simulink model "EstimateLaneCenter"  (R2024a)
settings: configuration reference "csMultiInstance" (kept outside this file)
undefined symbols (not defined in the file or in its folder): HalfLaneWidth, Ts
Description:
  | Model to esitmate centerline of the lane from information about the lane boundaries.
settings Model: DataDictionary=DD_EstimateLaneCenter.sldd  EnableAccessToBaseWorkspace=off  Creator=The MathWorks, Inc.  LastModifiedBy=The MathWorks, Inc.
settings ConfigSetRef: SourceName=csMultiInstance

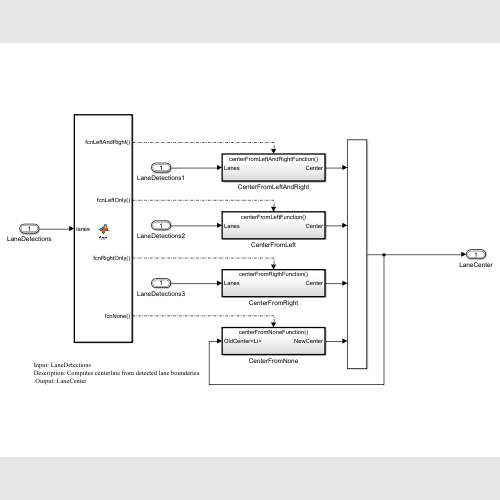
[thumbnail: Simulink's stored preview of the top-level diagram]
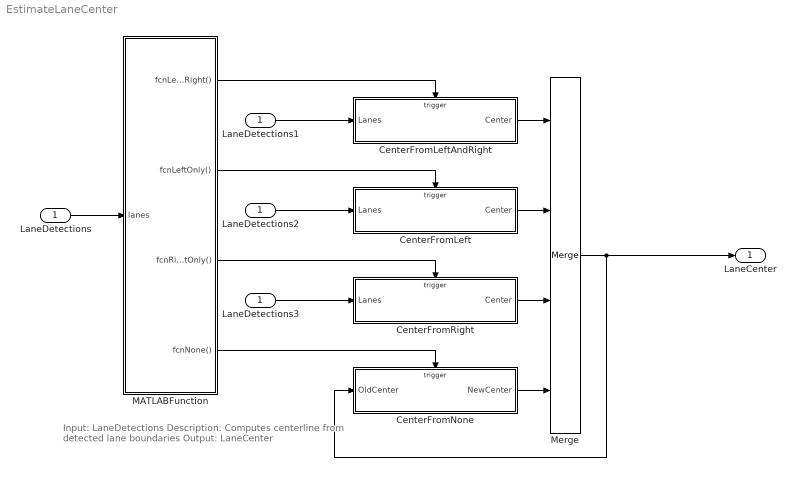
== system EstimateLaneCenter ==
  note: Input: LaneDetections
      | Description: Computes centerline from detected lane boundaries
      | Output: LaneCenter
  LaneDetections : Inport  OutDataTypeStr=Bus: LaneSensor  PortDimensions=1  SampleTime=Ts
  CenterFromLeft : Subsystem  TreatAsAtomicUnit=on
  CenterFromLeftAndRight : Subsystem  TreatAsAtomicUnit=on
  CenterFromNone : Subsystem  TreatAsAtomicUnit=on
  CenterFromRight : Subsystem  TreatAsAtomicUnit=on
  LaneDetections1 : InportShadow  OutDataTypeStr=Bus: LaneSensor  PortDimensions=1  SampleTime=Ts
  LaneDetections2 : InportShadow  OutDataTypeStr=Bus: LaneSensor  PortDimensions=1  SampleTime=Ts
  LaneDetections3 : InportShadow  OutDataTypeStr=Bus: LaneSensor  PortDimensions=1  SampleTime=Ts
  MATLABFunction : MATLAB Function  TreatAsAtomicUnit=on
  Merge : Merge  Inputs=4
  LaneCenter : Outport  OutDataTypeStr=Bus: BusLaneCenter  PortDimensions=1  SampleTime=Ts
  wires:
  MATLABFunction/1(fcnLeftAndRight()) -> CenterFromLeftAndRight/Trigger
  CenterFromNone/1(NewCenter) -> Merge/4
  MATLABFunction/3(fcnRightOnly()) -> CenterFromRight/Trigger
  CenterFromLeft/1(Center) -> Merge/2
  LaneDetections/1 -> MATLABFunction/1(lanes)
  MATLABFunction/4(fcnNone()) -> CenterFromNone/Trigger
  MATLABFunction/2(fcnLeftOnly()) -> CenterFromLeft/Trigger
  CenterFromRight/1(Center) -> Merge/3
  CenterFromLeftAndRight/1(Center) -> Merge/1
  LaneDetections1/1 -> CenterFromLeftAndRight/1(Lanes)
  LaneDetections3/1 -> CenterFromRight/1(Lanes)
  LaneDetections2/1 -> CenterFromLeft/1(Lanes)
  Merge/1 -> LaneCenter/1, CenterFromNone/1(OldCenter)

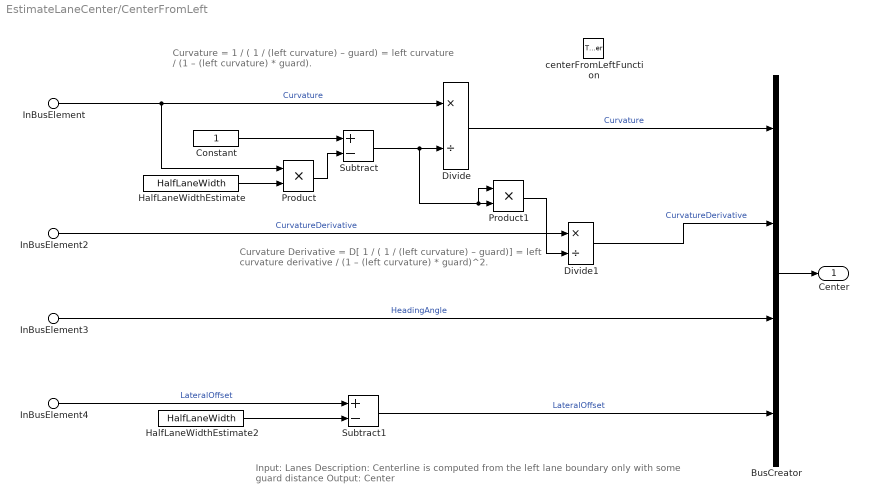
== system EstimateLaneCenter/CenterFromLeft ==
  note: Curvature Derivative
      | = D[ 1 / ( 1 / (left curvature) – guard)]
      | = left curvature derivative / (1 – (left curvature) * guard)^2.
  note: Curvature
      | = 1 / ( 1 / (left curvature) – guard)
      | = left curvature / (1 – (left curvature) * guard).
  note: Input: Lanes
      | Description: Centerline is computed from the left lane boundary only with some guard distance
      | Output: Center
  InBusElement : Inport  PortName=Lanes  Element=Left.Curvature
  InBusElement2 : Inport  PortName=Lanes  Element=Left.CurvatureDerivative
  InBusElement3 : Inport  PortName=Lanes  Element=Left.HeadingAngle
  InBusElement4 : Inport  PortName=Lanes  Element=Left.LateralOffset
  centerFromLeftFunction : TriggerPort  TriggerType=function-call  VariantControl=Variant
  BusCreator : BusCreator  Inputs=4
  Constant : Constant  OutDataTypeStr=single
  Divide : Product  Inputs=*/
  Divide1 : Product  Inputs=*/
  HalfLaneWidthEstimate : Constant  Value=HalfLaneWidth  OutDataTypeStr=single
  HalfLaneWidthEstimate2 : Constant  Value=HalfLaneWidth  OutDataTypeStr=single
  Product : Product
  Product1 : Product
  Subtract : Sum  Inputs=+-
  Subtract1 : Sum  Inputs=+-
  Center : Outport  VectorParamsAs1DForOutWhenUnconnected=off
  wires:
  BusCreator/1 -> Center/1
  Divide1/1 -> BusCreator/2  "CurvatureDerivative"
  Divide/1 -> BusCreator/1  "Curvature"
  InBusElement3/1 -> BusCreator/3  "HeadingAngle"
  Subtract1/1 -> BusCreator/4  "LateralOffset"
  InBusElement/1 -> Product/1, Divide/1  "Curvature"
  Subtract/1 -> Product1/1, Product1/2, Divide/2
  HalfLaneWidthEstimate/1 -> Product/2
  Constant/1 -> Subtract/1
  InBusElement4/1 -> Subtract1/1  "LateralOffset"
  HalfLaneWidthEstimate2/1 -> Subtract1/2
  Product/1 -> Subtract/2
  Product1/1 -> Divide1/2
  InBusElement2/1 -> Divide1/1  "CurvatureDerivative"

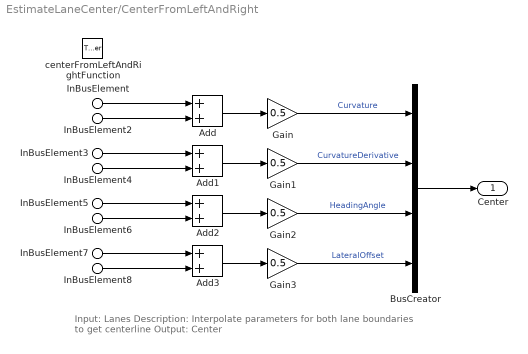
== system EstimateLaneCenter/CenterFromLeftAndRight ==
  note: Input: Lanes
      | Description: Interpolate parameters for both lane boundaries to get centerline
      | Output: Center
  InBusElement : Inport  PortName=Lanes  Element=Left.Curvature
  InBusElement3 : Inport  PortName=Lanes  Element=Left.CurvatureDerivative
  InBusElement5 : Inport  PortName=Lanes  Element=Left.HeadingAngle
  InBusElement7 : Inport  PortName=Lanes  Element=Left.LateralOffset
  InBusElement2 : Inport  PortName=Lanes  Element=Right.Curvature
  InBusElement4 : Inport  PortName=Lanes  Element=Right.CurvatureDerivative
  InBusElement6 : Inport  PortName=Lanes  Element=Right.HeadingAngle
  InBusElement8 : Inport  PortName=Lanes  Element=Right.LateralOffset
  centerFromLeftAndRightFunction : TriggerPort  TriggerType=function-call  VariantControl=Variant
  Add{,1..3} (4 alike) : Sum
  BusCreator : BusCreator  Inputs=4
  Gain{,1..3} (4 alike) : Gain  Gain=0.5
  Center : Outport  VectorParamsAs1DForOutWhenUnconnected=off
  wires:
  Add/1 -> Gain/1
  Gain/1 -> BusCreator/1  "Curvature"
  Add1/1 -> Gain1/1
  Gain1/1 -> BusCreator/2  "CurvatureDerivative"
  Add2/1 -> Gain2/1
  Gain2/1 -> BusCreator/3  "HeadingAngle"
  Add3/1 -> Gain3/1
  Gain3/1 -> BusCreator/4  "LateralOffset"
  BusCreator/1 -> Center/1
  InBusElement/1 -> Add/1
  InBusElement2/1 -> Add/2
  InBusElement3/1 -> Add1/1
  InBusElement4/1 -> Add1/2
  InBusElement5/1 -> Add2/1
  InBusElement6/1 -> Add2/2
  InBusElement8/1 -> Add3/2
  InBusElement7/1 -> Add3/1

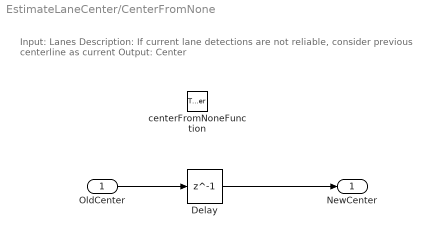
== system EstimateLaneCenter/CenterFromNone ==
  note: Input: Lanes
      | Description: If current lane detections are not reliable, consider previous centerline as current
      | Output: Center
  OldCenter : Inport
      settings: LatchInputForFeedbackSignals=on
  centerFromNoneFunction : TriggerPort  TriggerType=function-call  VariantControl=Variant
  Delay : Delay  DelayLength=1
  NewCenter : Outport  VectorParamsAs1DForOutWhenUnconnected=off
  wires:
  OldCenter/1 -> Delay/1
  Delay/1 -> NewCenter/1

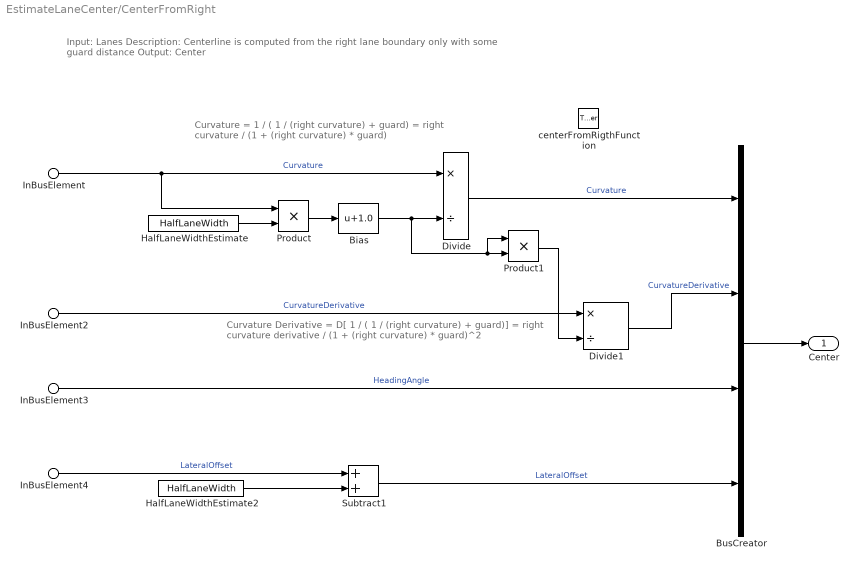
== system EstimateLaneCenter/CenterFromRight ==
  note: Curvature
      | = 1 / ( 1 / (right curvature) + guard)
      | = right curvature / (1 + (right curvature) * guard)
  note: Curvature Derivative
      | = D[ 1 / ( 1 / (right curvature) + guard)]
      | = right curvature derivative / (1 + (right curvature) * guard)^2
  note: Input: Lanes
      | Description: Centerline is computed from the right lane boundary only with some guard distance
      | Output: Center
  InBusElement : Inport  PortName=Lanes  Element=Right.Curvature
  InBusElement2 : Inport  PortName=Lanes  Element=Right.CurvatureDerivative
  InBusElement3 : Inport  PortName=Lanes  Element=Right.HeadingAngle
  InBusElement4 : Inport  PortName=Lanes  Element=Right.LateralOffset
  centerFromRigthFunction : TriggerPort  TriggerType=function-call  VariantControl=Variant
  Bias : Bias  Bias=1.0  SaturateOnIntegerOverflow=off
  BusCreator : BusCreator  Inputs=4  OutDataTypeStr=Bus: BusLaneCenter
  Divide : Product  Inputs=*/
  Divide1 : Product  Inputs=*/
  HalfLaneWidthEstimate : Constant  Value=HalfLaneWidth  OutDataTypeStr=single
  HalfLaneWidthEstimate2 : Constant  Value=HalfLaneWidth  OutDataTypeStr=single
  Product : Product
  Product1 : Product
  Subtract1 : Sum
  Center : Outport  VectorParamsAs1DForOutWhenUnconnected=off
  wires:
  Divide1/1 -> BusCreator/2  "CurvatureDerivative"
  InBusElement3/1 -> BusCreator/3  "HeadingAngle"
  HalfLaneWidthEstimate2/1 -> Subtract1/2
  InBusElement4/1 -> Subtract1/1  "LateralOffset"
  Divide/1 -> BusCreator/1  "Curvature"
  Subtract1/1 -> BusCreator/4  "LateralOffset"
  BusCreator/1 -> Center/1
  InBusElement/1 -> Product/1, Divide/1  "Curvature"
  Product/1 -> Bias/1
  HalfLaneWidthEstimate/1 -> Product/2
  Bias/1 -> Product1/1, Product1/2, Divide/2
  InBusElement2/1 -> Divide1/1  "CurvatureDerivative"
  Product1/1 -> Divide1/2

== matlab function EstimateLaneCenter/MATLABFunction ==
  data: lanes input Bus: LaneSensor size=1
  events: fcnLeftAndRight output FUNCTION_CALL_EVENT; fcnLeftOnly output FUNCTION_CALL_EVENT; fcnRightOnly output FUNCTION_CALL_EVENT; fcnNone output FUNCTION_CALL_EVENT
function fcn(lanes)
% FUNCTION NAME:
%   fcn
%
% DESCRIPTION:
%   checks the strength for each lane boundary, and
%	triggers an appropriate function accordingly.
%
% INPUT:
%   lanes - (LaneSensor) output of the lane sensor
%
% OUTPUT:
%   None
%
% ASSUMPTIONS AND LIMITATIONS:
%   None
%

%   Copyright 1984-2020 The MathWorks, Inc. 

leftStrength  = lanes.Left.Strength;
rightStrength = lanes.Right.Strength;

strengthThreshold = single(0);

if (leftStrength > strengthThreshold) && (rightStrength > strengthThreshold)
   fcnLeftAndRight();

elseif leftStrength > strengthThreshold
    fcnLeftOnly();

elseif rightStrength > strengthThreshold
    fcnRightOnly();

else
    fcnNone();
end
